simulink model "RudderOpenLoopResponse"  (R2021a)
settings: Solver=VariableStepAuto  StartTime=0.0  StopTime=60  RelTol=1e-3
values from neighbouring files (symbols this model uses):
  v = sqrt(mass * g / lift_b)    [setup.m]
undefined symbols (not defined in the file or in its folder): I_zz, rudder_m
libraries: simulink_extras x1
settings Model: Creator=amaar  LastModifiedBy=amaar

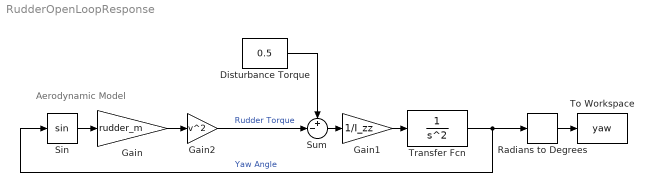
== system RudderOpenLoopResponse ==
  note: Aerodynamic Model
  Disturbance Torque : Constant  Value=0.5
  Gain : Gain  Gain=rudder_m
  Gain1 : Gain  Gain=1/I_zz
  Gain2 : Gain  Gain=v^2
  Radians to Degrees : simulink_extras/Transformations/Radians to Degrees
  Sin : Trigonometry
  Sum : Sum  Inputs=+-|
  To Workspace : ToWorkspace  VariableName=yaw  SaveFormat=Timeseries  SampleTime=-1
  Transfer Fcn : TransferFcn  Denominator=[1 0 0]
  wires:
  Transfer Fcn/1 -> Radians to Degrees/1, Sin/1  "Yaw Angle"
  Gain2/1 -> Sum/2  "Rudder Torque"
  Sum/1 -> Gain1/1
  Disturbance Torque/1 -> Sum/1
  Gain1/1 -> Transfer Fcn/1
  Gain/1 -> Gain2/1
  Sin/1 -> Gain/1
  Radians to Degrees/1 -> To Workspace/1
